simulink model "untuned_filter"  (R2021a)
settings: Solver=VariableStepAuto  StartTime=0.0  StopTime=10.0  RelTol=1e-3
libraries: xbsIndex_r4 x753
(part 2 of 2)

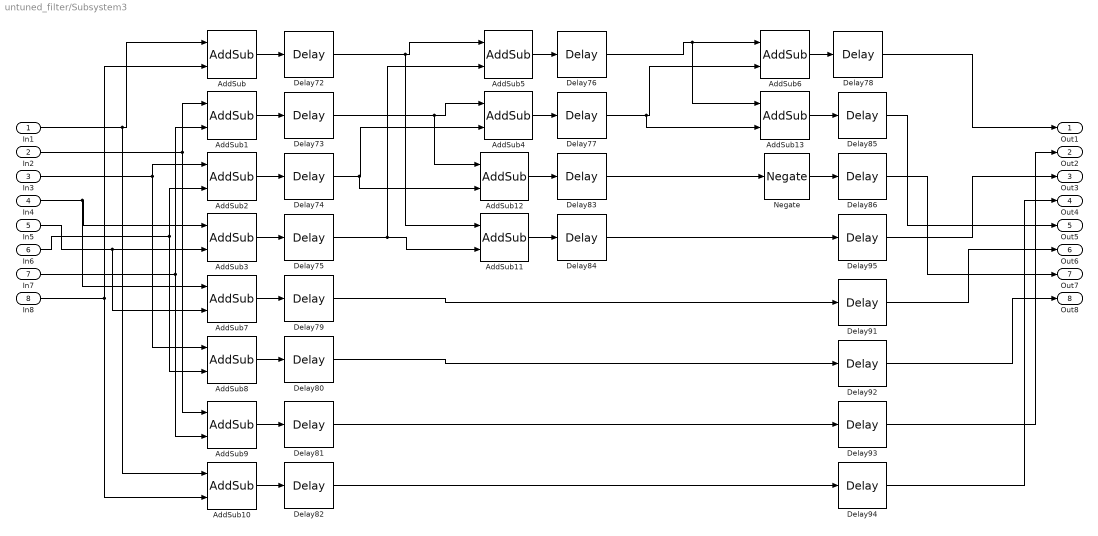
== system untuned_filter/Subsystem3 ==
  In1 : Inport
  In2 : Inport  Port=2
  In3 : Inport  Port=3
  In4 : Inport  Port=4
  In5 : Inport  Port=5
  In6 : Inport  Port=6
  In7 : Inport  Port=7
  In8 : Inport  Port=8
  AddSub{,1..6} (7 alike) : xbsIndex_r4/AddSub  mode=Addition  use_carryin=off  use_carryout=off  en=off  latency=0  precision=User Defined  arith_type="Signed  (2's comp)"  n_bits=Wa  bin_pt=Da  quantization="Round  (unbiased: +/- Inf)"  overflow=Saturate  use_behavioral_HDL=off  hw_selection=Fabric  pipelined=off  dbl_ovrd=off  block_type=addsub
  AddSub{7..13} (7 alike) : xbsIndex_r4/AddSub  mode=Subtraction  use_carryin=off  use_carryout=off  en=off  latency=0  precision=User Defined  arith_type="Signed  (2's comp)"  n_bits=Wa  bin_pt=Da  quantization="Round  (unbiased: +/- Inf)"  overflow=Saturate  use_behavioral_HDL=off  hw_selection=Fabric  pipelined=off  dbl_ovrd=off  block_type=addsub
  Delay{72..86,91..95} (20 alike) : xbsIndex_r4/Delay  rst=off  infoeditControl=Selection of Reset will increase slice count due to use of real FFs and instead of SRLs  en=off  latency=1  reg_retiming=off  dbl_ovrd=off  block_type=delay
  Negate : xbsIndex_r4/Negate  precision=User Defined  arith_type="Signed  (2's comp)"  n_bits=Wa  bin_pt=Da  quantization="Round  (unbiased: +/- Inf)"  overflow=Saturate  en=off  latency=0  dbl_ovrd=off  block_type=negate
  Out1 : Outport
  Out2 : Outport  Port=2
  Out3 : Outport  Port=3
  Out4 : Outport  Port=4
  Out5 : Outport  Port=5
  Out6 : Outport  Port=6
  Out7 : Outport  Port=7
  Out8 : Outport  Port=8
  wires:
  Delay86/1 -> Out7/1
  In5/1 -> AddSub7/2, AddSub3/2
  Negate/1 -> Delay86/1
  Delay74/1 -> AddSub12/2, AddSub4/2
  In8/1 -> AddSub/2, AddSub10/2
  In7/1 -> AddSub1/2, AddSub9/2
  Delay82/1 -> Delay94/1
  AddSub2/1 -> Delay74/1
  Delay84/1 -> Delay95/1
  Delay80/1 -> Delay92/1
  AddSub8/1 -> Delay80/1
  Delay76/1 -> AddSub13/1, AddSub6/1
  Delay77/1 -> AddSub13/2, AddSub6/2
  Delay92/1 -> Out8/1
  Delay72/1 -> AddSub11/1, AddSub5/1
  Delay73/1 -> AddSub12/1, AddSub4/1
  AddSub9/1 -> Delay81/1
  In6/1 -> AddSub2/2, AddSub8/2
  In4/1 -> AddSub7/1, AddSub3/1
  In3/1 -> AddSub2/1, AddSub8/1
  Delay79/1 -> Delay91/1
  In1/1 -> AddSub10/1, AddSub/1
  AddSub6/1 -> Delay78/1
  AddSub7/1 -> Delay79/1
  Delay83/1 -> Negate/1
  AddSub3/1 -> Delay75/1
  AddSub13/1 -> Delay85/1
  In2/1 -> AddSub1/1, AddSub9/1
  Delay91/1 -> Out6/1
  Delay75/1 -> AddSub5/2, AddSub11/2
  AddSub10/1 -> Delay82/1
  AddSub12/1 -> Delay83/1
  AddSub11/1 -> Delay84/1
  AddSub5/1 -> Delay76/1
  Delay78/1 -> Out1/1
  AddSub4/1 -> Delay77/1
  Delay81/1 -> Delay93/1
  AddSub1/1 -> Delay73/1
  AddSub/1 -> Delay72/1
  Delay95/1 -> Out3/1
  Delay94/1 -> Out4/1
  Delay85/1 -> Out5/1
  Delay93/1 -> Out2/1

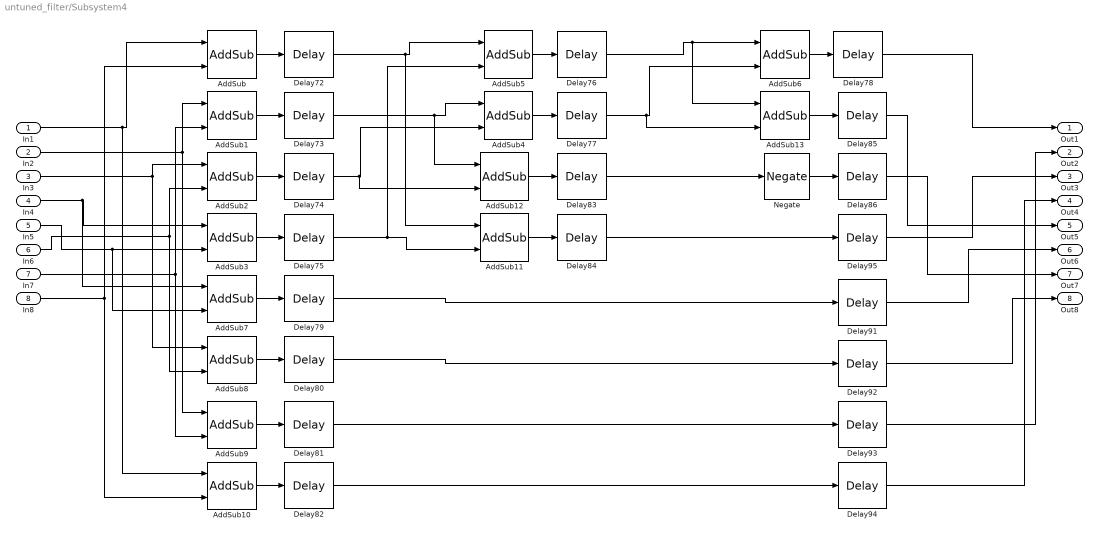
== system untuned_filter/Subsystem4 ==
  In1 : Inport
  In2 : Inport  Port=2
  In3 : Inport  Port=3
  In4 : Inport  Port=4
  In5 : Inport  Port=5
  In6 : Inport  Port=6
  In7 : Inport  Port=7
  In8 : Inport  Port=8
  AddSub{,1..6} (7 alike) : xbsIndex_r4/AddSub  mode=Addition  use_carryin=off  use_carryout=off  en=off  latency=0  precision=User Defined  arith_type="Signed  (2's comp)"  n_bits=Wa  bin_pt=Da  quantization="Round  (unbiased: +/- Inf)"  overflow=Saturate  use_behavioral_HDL=off  hw_selection=Fabric  pipelined=off  dbl_ovrd=off  block_type=addsub
  AddSub{7..13} (7 alike) : xbsIndex_r4/AddSub  mode=Subtraction  use_carryin=off  use_carryout=off  en=off  latency=0  precision=User Defined  arith_type="Signed  (2's comp)"  n_bits=Wa  bin_pt=Da  quantization="Round  (unbiased: +/- Inf)"  overflow=Saturate  use_behavioral_HDL=off  hw_selection=Fabric  pipelined=off  dbl_ovrd=off  block_type=addsub
  Delay{72..86,91..95} (20 alike) : xbsIndex_r4/Delay  rst=off  infoeditControl=Selection of Reset will increase slice count due to use of real FFs and instead of SRLs  en=off  latency=1  reg_retiming=off  dbl_ovrd=off  block_type=delay
  Negate : xbsIndex_r4/Negate  precision=User Defined  arith_type="Signed  (2's comp)"  n_bits=Wa  bin_pt=Da  quantization="Round  (unbiased: +/- Inf)"  overflow=Saturate  en=off  latency=0  dbl_ovrd=off  block_type=negate
  Out1 : Outport
  Out2 : Outport  Port=2
  Out3 : Outport  Port=3
  Out4 : Outport  Port=4
  Out5 : Outport  Port=5
  Out6 : Outport  Port=6
  Out7 : Outport  Port=7
  Out8 : Outport  Port=8
  wires:
  Delay86/1 -> Out7/1
  In5/1 -> AddSub7/2, AddSub3/2
  Negate/1 -> Delay86/1
  Delay74/1 -> AddSub12/2, AddSub4/2
  In8/1 -> AddSub/2, AddSub10/2
  In7/1 -> AddSub1/2, AddSub9/2
  Delay82/1 -> Delay94/1
  AddSub2/1 -> Delay74/1
  Delay84/1 -> Delay95/1
  Delay80/1 -> Delay92/1
  AddSub8/1 -> Delay80/1
  Delay76/1 -> AddSub13/1, AddSub6/1
  Delay77/1 -> AddSub13/2, AddSub6/2
  Delay92/1 -> Out8/1
  Delay72/1 -> AddSub11/1, AddSub5/1
  Delay73/1 -> AddSub12/1, AddSub4/1
  AddSub9/1 -> Delay81/1
  In6/1 -> AddSub2/2, AddSub8/2
  In4/1 -> AddSub7/1, AddSub3/1
  In3/1 -> AddSub2/1, AddSub8/1
  Delay79/1 -> Delay91/1
  In1/1 -> AddSub10/1, AddSub/1
  AddSub6/1 -> Delay78/1
  AddSub7/1 -> Delay79/1
  Delay83/1 -> Negate/1
  AddSub3/1 -> Delay75/1
  AddSub13/1 -> Delay85/1
  In2/1 -> AddSub1/1, AddSub9/1
  Delay91/1 -> Out6/1
  Delay75/1 -> AddSub5/2, AddSub11/2
  AddSub10/1 -> Delay82/1
  AddSub12/1 -> Delay83/1
  AddSub11/1 -> Delay84/1
  AddSub5/1 -> Delay76/1
  Delay78/1 -> Out1/1
  AddSub4/1 -> Delay77/1
  Delay81/1 -> Delay93/1
  AddSub1/1 -> Delay73/1
  AddSub/1 -> Delay72/1
  Delay95/1 -> Out3/1
  Delay94/1 -> Out4/1
  Delay85/1 -> Out5/1
  Delay93/1 -> Out2/1

== system untuned_filter/Subsystem5 ==
  In1 : Inport
  In2 : Inport  Port=2
  In3 : Inport  Port=3
  In4 : Inport  Port=4
  In5 : Inport  Port=5
  In6 : Inport  Port=6
  In7 : Inport  Port=7
  In8 : Inport  Port=8
  AddSub{,1..6} (7 alike) : xbsIndex_r4/AddSub  mode=Addition  use_carryin=off  use_carryout=off  en=off  latency=0  precision=User Defined  arith_type="Signed  (2's comp)"  n_bits=Wa  bin_pt=Da  quantization="Round  (unbiased: +/- Inf)"  overflow=Saturate  use_behavioral_HDL=off  hw_selection=Fabric  pipelined=off  dbl_ovrd=off  block_type=addsub
  AddSub{7..13} (7 alike) : xbsIndex_r4/AddSub  mode=Subtraction  use_carryin=off  use_carryout=off  en=off  latency=0  precision=User Defined  arith_type="Signed  (2's comp)"  n_bits=Wa  bin_pt=Da  quantization="Round  (unbiased: +/- Inf)"  overflow=Saturate  use_behavioral_HDL=off  hw_selection=Fabric  pipelined=off  dbl_ovrd=off  block_type=addsub
  Delay{72..86,91..95} (20 alike) : xbsIndex_r4/Delay  rst=off  infoeditControl=Selection of Reset will increase slice count due to use of real FFs and instead of SRLs  en=off  latency=1  reg_retiming=off  dbl_ovrd=off  block_type=delay
  Negate : xbsIndex_r4/Negate  precision=User Defined  arith_type="Signed  (2's comp)"  n_bits=Wa  bin_pt=Da  quantization="Round  (unbiased: +/- Inf)"  overflow=Saturate  en=off  latency=0  dbl_ovrd=off  block_type=negate
  Out1 : Outport
  Out2 : Outport  Port=2
  Out3 : Outport  Port=3
  Out4 : Outport  Port=4
  Out5 : Outport  Port=5
  Out6 : Outport  Port=6
  Out7 : Outport  Port=7
  Out8 : Outport  Port=8
  wires:
  Delay86/1 -> Out7/1
  In5/1 -> AddSub7/2, AddSub3/2
  Negate/1 -> Delay86/1
  Delay74/1 -> AddSub12/2, AddSub4/2
  In8/1 -> AddSub/2, AddSub10/2
  In7/1 -> AddSub1/2, AddSub9/2
  Delay82/1 -> Delay94/1
  AddSub2/1 -> Delay74/1
  Delay84/1 -> Delay95/1
  Delay80/1 -> Delay92/1
  AddSub8/1 -> Delay80/1
  Delay76/1 -> AddSub13/1, AddSub6/1
  Delay77/1 -> AddSub13/2, AddSub6/2
  Delay92/1 -> Out8/1
  Delay72/1 -> AddSub11/1, AddSub5/1
  Delay73/1 -> AddSub12/1, AddSub4/1
  AddSub9/1 -> Delay81/1
  In6/1 -> AddSub2/2, AddSub8/2
  In4/1 -> AddSub7/1, AddSub3/1
  In3/1 -> AddSub2/1, AddSub8/1
  Delay79/1 -> Delay91/1
  In1/1 -> AddSub10/1, AddSub/1
  AddSub6/1 -> Delay78/1
  AddSub7/1 -> Delay79/1
  Delay83/1 -> Negate/1
  AddSub3/1 -> Delay75/1
  AddSub13/1 -> Delay85/1
  In2/1 -> AddSub1/1, AddSub9/1
  Delay91/1 -> Out6/1
  Delay75/1 -> AddSub5/2, AddSub11/2
  AddSub10/1 -> Delay82/1
  AddSub12/1 -> Delay83/1
  AddSub11/1 -> Delay84/1
  AddSub5/1 -> Delay76/1
  Delay78/1 -> Out1/1
  AddSub4/1 -> Delay77/1
  Delay81/1 -> Delay93/1
  AddSub1/1 -> Delay73/1
  AddSub/1 -> Delay72/1
  Delay95/1 -> Out3/1
  Delay94/1 -> Out4/1
  Delay85/1 -> Out5/1
  Delay93/1 -> Out2/1

== system untuned_filter/Subsystem6 ==
  In1 : Inport
  In2 : Inport  Port=2
  In3 : Inport  Port=3
  In4 : Inport  Port=4
  In5 : Inport  Port=5
  In6 : Inport  Port=6
  In7 : Inport  Port=7
  In8 : Inport  Port=8
  AddSub{,1..6} (7 alike) : xbsIndex_r4/AddSub  mode=Addition  use_carryin=off  use_carryout=off  en=off  latency=0  precision=User Defined  arith_type="Signed  (2's comp)"  n_bits=Wa  bin_pt=Da  quantization="Round  (unbiased: +/- Inf)"  overflow=Saturate  use_behavioral_HDL=off  hw_selection=Fabric  pipelined=off  dbl_ovrd=off  block_type=addsub
  AddSub{7..13} (7 alike) : xbsIndex_r4/AddSub  mode=Subtraction  use_carryin=off  use_carryout=off  en=off  latency=0  precision=User Defined  arith_type="Signed  (2's comp)"  n_bits=Wa  bin_pt=Da  quantization="Round  (unbiased: +/- Inf)"  overflow=Saturate  use_behavioral_HDL=off  hw_selection=Fabric  pipelined=off  dbl_ovrd=off  block_type=addsub
  Delay{72..86,91..95} (20 alike) : xbsIndex_r4/Delay  rst=off  infoeditControl=Selection of Reset will increase slice count due to use of real FFs and instead of SRLs  en=off  latency=1  reg_retiming=off  dbl_ovrd=off  block_type=delay
  Negate : xbsIndex_r4/Negate  precision=User Defined  arith_type="Signed  (2's comp)"  n_bits=Wa  bin_pt=Da  quantization="Round  (unbiased: +/- Inf)"  overflow=Saturate  en=off  latency=0  dbl_ovrd=off  block_type=negate
  Out1 : Outport
  Out2 : Outport  Port=2
  Out3 : Outport  Port=3
  Out4 : Outport  Port=4
  Out5 : Outport  Port=5
  Out6 : Outport  Port=6
  Out7 : Outport  Port=7
  Out8 : Outport  Port=8
  wires:
  Delay86/1 -> Out7/1
  In5/1 -> AddSub7/2, AddSub3/2
  Negate/1 -> Delay86/1
  Delay74/1 -> AddSub12/2, AddSub4/2
  In8/1 -> AddSub/2, AddSub10/2
  In7/1 -> AddSub1/2, AddSub9/2
  Delay82/1 -> Delay94/1
  AddSub2/1 -> Delay74/1
  Delay84/1 -> Delay95/1
  Delay80/1 -> Delay92/1
  AddSub8/1 -> Delay80/1
  Delay76/1 -> AddSub13/1, AddSub6/1
  Delay77/1 -> AddSub13/2, AddSub6/2
  Delay92/1 -> Out8/1
  Delay72/1 -> AddSub11/1, AddSub5/1
  Delay73/1 -> AddSub12/1, AddSub4/1
  AddSub9/1 -> Delay81/1
  In6/1 -> AddSub2/2, AddSub8/2
  In4/1 -> AddSub7/1, AddSub3/1
  In3/1 -> AddSub2/1, AddSub8/1
  Delay79/1 -> Delay91/1
  In1/1 -> AddSub10/1, AddSub/1
  AddSub6/1 -> Delay78/1
  AddSub7/1 -> Delay79/1
  Delay83/1 -> Negate/1
  AddSub3/1 -> Delay75/1
  AddSub13/1 -> Delay85/1
  In2/1 -> AddSub1/1, AddSub9/1
  Delay91/1 -> Out6/1
  Delay75/1 -> AddSub5/2, AddSub11/2
  AddSub10/1 -> Delay82/1
  AddSub12/1 -> Delay83/1
  AddSub11/1 -> Delay84/1
  AddSub5/1 -> Delay76/1
  Delay78/1 -> Out1/1
  AddSub4/1 -> Delay77/1
  Delay81/1 -> Delay93/1
  AddSub1/1 -> Delay73/1
  AddSub/1 -> Delay72/1
  Delay95/1 -> Out3/1
  Delay94/1 -> Out4/1
  Delay85/1 -> Out5/1
  Delay93/1 -> Out2/1

== system untuned_filter/Subsystem7 ==
  In1 : Inport
  In2 : Inport  Port=2
  In3 : Inport  Port=3
  In4 : Inport  Port=4
  In5 : Inport  Port=5
  In6 : Inport  Port=6
  In7 : Inport  Port=7
  In8 : Inport  Port=8
  AddSub{,1..6} (7 alike) : xbsIndex_r4/AddSub  mode=Addition  use_carryin=off  use_carryout=off  en=off  latency=0  precision=User Defined  arith_type="Signed  (2's comp)"  n_bits=Wa  bin_pt=Da  quantization="Round  (unbiased: +/- Inf)"  overflow=Saturate  use_behavioral_HDL=off  hw_selection=Fabric  pipelined=off  dbl_ovrd=off  block_type=addsub
  AddSub{7..13} (7 alike) : xbsIndex_r4/AddSub  mode=Subtraction  use_carryin=off  use_carryout=off  en=off  latency=0  precision=User Defined  arith_type="Signed  (2's comp)"  n_bits=Wa  bin_pt=Da  quantization="Round  (unbiased: +/- Inf)"  overflow=Saturate  use_behavioral_HDL=off  hw_selection=Fabric  pipelined=off  dbl_ovrd=off  block_type=addsub
  Delay{72..86,91..95} (20 alike) : xbsIndex_r4/Delay  rst=off  infoeditControl=Selection of Reset will increase slice count due to use of real FFs and instead of SRLs  en=off  latency=1  reg_retiming=off  dbl_ovrd=off  block_type=delay
  Negate : xbsIndex_r4/Negate  precision=User Defined  arith_type="Signed  (2's comp)"  n_bits=Wa  bin_pt=Da  quantization="Round  (unbiased: +/- Inf)"  overflow=Saturate  en=off  latency=0  dbl_ovrd=off  block_type=negate
  Out1 : Outport
  Out2 : Outport  Port=2
  Out3 : Outport  Port=3
  Out4 : Outport  Port=4
  Out5 : Outport  Port=5
  Out6 : Outport  Port=6
  Out7 : Outport  Port=7
  Out8 : Outport  Port=8
  wires:
  Delay86/1 -> Out7/1
  In5/1 -> AddSub7/2, AddSub3/2
  Negate/1 -> Delay86/1
  Delay74/1 -> AddSub12/2, AddSub4/2
  In8/1 -> AddSub/2, AddSub10/2
  In7/1 -> AddSub1/2, AddSub9/2
  Delay82/1 -> Delay94/1
  AddSub2/1 -> Delay74/1
  Delay84/1 -> Delay95/1
  Delay80/1 -> Delay92/1
  AddSub8/1 -> Delay80/1
  Delay76/1 -> AddSub13/1, AddSub6/1
  Delay77/1 -> AddSub13/2, AddSub6/2
  Delay92/1 -> Out8/1
  Delay72/1 -> AddSub11/1, AddSub5/1
  Delay73/1 -> AddSub12/1, AddSub4/1
  AddSub9/1 -> Delay81/1
  In6/1 -> AddSub2/2, AddSub8/2
  In4/1 -> AddSub7/1, AddSub3/1
  In3/1 -> AddSub2/1, AddSub8/1
  Delay79/1 -> Delay91/1
  In1/1 -> AddSub10/1, AddSub/1
  AddSub6/1 -> Delay78/1
  AddSub7/1 -> Delay79/1
  Delay83/1 -> Negate/1
  AddSub3/1 -> Delay75/1
  AddSub13/1 -> Delay85/1
  In2/1 -> AddSub1/1, AddSub9/1
  Delay91/1 -> Out6/1
  Delay75/1 -> AddSub5/2, AddSub11/2
  AddSub10/1 -> Delay82/1
  AddSub12/1 -> Delay83/1
  AddSub11/1 -> Delay84/1
  AddSub5/1 -> Delay76/1
  Delay78/1 -> Out1/1
  AddSub4/1 -> Delay77/1
  Delay81/1 -> Delay93/1
  AddSub1/1 -> Delay73/1
  AddSub/1 -> Delay72/1
  Delay95/1 -> Out3/1
  Delay94/1 -> Out4/1
  Delay85/1 -> Out5/1
  Delay93/1 -> Out2/1

== system untuned_filter/Subsystem8 ==
  In1 : Inport
  In2 : Inport  Port=2
  In3 : Inport  Port=3
  In4 : Inport  Port=4
  In5 : Inport  Port=5
  In6 : Inport  Port=6
  In7 : Inport  Port=7
  In8 : Inport  Port=8
  AddSub{,1..6} (7 alike) : xbsIndex_r4/AddSub  mode=Addition  use_carryin=off  use_carryout=off  en=off  latency=0  precision=User Defined  arith_type="Signed  (2's comp)"  n_bits=Wa  bin_pt=Da  quantization="Round  (unbiased: +/- Inf)"  overflow=Saturate  use_behavioral_HDL=off  hw_selection=Fabric  pipelined=off  dbl_ovrd=off  block_type=addsub
  AddSub{7..13} (7 alike) : xbsIndex_r4/AddSub  mode=Subtraction  use_carryin=off  use_carryout=off  en=off  latency=0  precision=User Defined  arith_type="Signed  (2's comp)"  n_bits=Wa  bin_pt=Da  quantization="Round  (unbiased: +/- Inf)"  overflow=Saturate  use_behavioral_HDL=off  hw_selection=Fabric  pipelined=off  dbl_ovrd=off  block_type=addsub
  Delay{72..86,91..95} (20 alike) : xbsIndex_r4/Delay  rst=off  infoeditControl=Selection of Reset will increase slice count due to use of real FFs and instead of SRLs  en=off  latency=1  reg_retiming=off  dbl_ovrd=off  block_type=delay
  Negate : xbsIndex_r4/Negate  precision=User Defined  arith_type="Signed  (2's comp)"  n_bits=Wa  bin_pt=Da  quantization="Round  (unbiased: +/- Inf)"  overflow=Saturate  en=off  latency=0  dbl_ovrd=off  block_type=negate
  Out1 : Outport
  Out2 : Outport  Port=2
  Out3 : Outport  Port=3
  Out4 : Outport  Port=4
  Out5 : Outport  Port=5
  Out6 : Outport  Port=6
  Out7 : Outport  Port=7
  Out8 : Outport  Port=8
  wires:
  Delay86/1 -> Out7/1
  In5/1 -> AddSub7/2, AddSub3/2
  Negate/1 -> Delay86/1
  Delay74/1 -> AddSub12/2, AddSub4/2
  In8/1 -> AddSub/2, AddSub10/2
  In7/1 -> AddSub1/2, AddSub9/2
  Delay82/1 -> Delay94/1
  AddSub2/1 -> Delay74/1
  Delay84/1 -> Delay95/1
  Delay80/1 -> Delay92/1
  AddSub8/1 -> Delay80/1
  Delay76/1 -> AddSub13/1, AddSub6/1
  Delay77/1 -> AddSub13/2, AddSub6/2
  Delay92/1 -> Out8/1
  Delay72/1 -> AddSub11/1, AddSub5/1
  Delay73/1 -> AddSub12/1, AddSub4/1
  AddSub9/1 -> Delay81/1
  In6/1 -> AddSub2/2, AddSub8/2
  In4/1 -> AddSub7/1, AddSub3/1
  In3/1 -> AddSub2/1, AddSub8/1
  Delay79/1 -> Delay91/1
  In1/1 -> AddSub10/1, AddSub/1
  AddSub6/1 -> Delay78/1
  AddSub7/1 -> Delay79/1
  Delay83/1 -> Negate/1
  AddSub3/1 -> Delay75/1
  AddSub13/1 -> Delay85/1
  In2/1 -> AddSub1/1, AddSub9/1
  Delay91/1 -> Out6/1
  Delay75/1 -> AddSub5/2, AddSub11/2
  AddSub10/1 -> Delay82/1
  AddSub12/1 -> Delay83/1
  AddSub11/1 -> Delay84/1
  AddSub5/1 -> Delay76/1
  Delay78/1 -> Out1/1
  AddSub4/1 -> Delay77/1
  Delay81/1 -> Delay93/1
  AddSub1/1 -> Delay73/1
  AddSub/1 -> Delay72/1
  Delay95/1 -> Out3/1
  Delay94/1 -> Out4/1
  Delay85/1 -> Out5/1
  Delay93/1 -> Out2/1

== system untuned_filter/Subsystem9 ==
  In1 : Inport
  In2 : Inport  Port=2
  In3 : Inport  Port=3
  In4 : Inport  Port=4
  In5 : Inport  Port=5
  In6 : Inport  Port=6
  In7 : Inport  Port=7
  In8 : Inport  Port=8
  AddSub{,1..6} (7 alike) : xbsIndex_r4/AddSub  mode=Addition  use_carryin=off  use_carryout=off  en=off  latency=0  precision=User Defined  arith_type="Signed  (2's comp)"  n_bits=Wa  bin_pt=Da  quantization="Round  (unbiased: +/- Inf)"  overflow=Saturate  use_behavioral_HDL=off  hw_selection=Fabric  pipelined=off  dbl_ovrd=off  block_type=addsub
  AddSub{7..13} (7 alike) : xbsIndex_r4/AddSub  mode=Subtraction  use_carryin=off  use_carryout=off  en=off  latency=0  precision=User Defined  arith_type="Signed  (2's comp)"  n_bits=Wa  bin_pt=Da  quantization="Round  (unbiased: +/- Inf)"  overflow=Saturate  use_behavioral_HDL=off  hw_selection=Fabric  pipelined=off  dbl_ovrd=off  block_type=addsub
  Delay{72..86,91..95} (20 alike) : xbsIndex_r4/Delay  rst=off  infoeditControl=Selection of Reset will increase slice count due to use of real FFs and instead of SRLs  en=off  latency=1  reg_retiming=off  dbl_ovrd=off  block_type=delay
  Negate : xbsIndex_r4/Negate  precision=User Defined  arith_type="Signed  (2's comp)"  n_bits=Wa  bin_pt=Da  quantization="Round  (unbiased: +/- Inf)"  overflow=Saturate  en=off  latency=0  dbl_ovrd=off  block_type=negate
  Out1 : Outport
  Out2 : Outport  Port=2
  Out3 : Outport  Port=3
  Out4 : Outport  Port=4
  Out5 : Outport  Port=5
  Out6 : Outport  Port=6
  Out7 : Outport  Port=7
  Out8 : Outport  Port=8
  wires:
  Delay86/1 -> Out7/1
  In5/1 -> AddSub7/2, AddSub3/2
  Negate/1 -> Delay86/1
  Delay74/1 -> AddSub12/2, AddSub4/2
  In8/1 -> AddSub/2, AddSub10/2
  In7/1 -> AddSub1/2, AddSub9/2
  Delay82/1 -> Delay94/1
  AddSub2/1 -> Delay74/1
  Delay84/1 -> Delay95/1
  Delay80/1 -> Delay92/1
  AddSub8/1 -> Delay80/1
  Delay76/1 -> AddSub13/1, AddSub6/1
  Delay77/1 -> AddSub13/2, AddSub6/2
  Delay92/1 -> Out8/1
  Delay72/1 -> AddSub11/1, AddSub5/1
  Delay73/1 -> AddSub12/1, AddSub4/1
  AddSub9/1 -> Delay81/1
  In6/1 -> AddSub2/2, AddSub8/2
  In4/1 -> AddSub7/1, AddSub3/1
  In3/1 -> AddSub2/1, AddSub8/1
  Delay79/1 -> Delay91/1
  In1/1 -> AddSub10/1, AddSub/1
  AddSub6/1 -> Delay78/1
  AddSub7/1 -> Delay79/1
  Delay83/1 -> Negate/1
  AddSub3/1 -> Delay75/1
  AddSub13/1 -> Delay85/1
  In2/1 -> AddSub1/1, AddSub9/1
  Delay91/1 -> Out6/1
  Delay75/1 -> AddSub5/2, AddSub11/2
  AddSub10/1 -> Delay82/1
  AddSub12/1 -> Delay83/1
  AddSub11/1 -> Delay84/1
  AddSub5/1 -> Delay76/1
  Delay78/1 -> Out1/1
  AddSub4/1 -> Delay77/1
  Delay81/1 -> Delay93/1
  AddSub1/1 -> Delay73/1
  AddSub/1 -> Delay72/1
  Delay95/1 -> Out3/1
  Delay94/1 -> Out4/1
  Delay85/1 -> Out5/1
  Delay93/1 -> Out2/1
